simulink model "MS_CDM_substructure"  (R2022b)
settings: Solver=FixedStepAuto  StartTime=0.0  StopTime=55.0  FixedStep=0.001  RelTol=1e-3
values from neighbouring files (symbols this model uses):
  a_ps = K_ps - (2 * M_ps) / (dt)^2    (= -21398788.6)    [Final_10DOFs_RTHS.m]    (also in ThreeDOFs_CDM_substructure.m = -1999400; structure_2DOFs.m = -9.988)
  ACC_el = ACC_el(1:10000,:)    [ThreeDOFs_Dampling.m]    (also in ThreeDOFs_noDampling.m; multiDOFs_CDM_highspeed_Dampling.m = ACC_el(1:2000,:); multiDOFs_auto_for_loop.m = ACC_el(1:1000,:); multiDOFs_highspeed.m = ACC_el(1:1000,:))
  an = Kn - (2 * Mn) / (dt)^2    [Final_10DOFs_RTHS.m]    (also in ThreeDOFs_CDM_Dampling.m; multiDOFs_CDM_highspeed_Dampling.m; test.m)
  b_ps = M_ps / dt^2 - C_ps / (2*dt)    (= 10684932)    [Final_10DOFs_RTHS.m]    (also in ThreeDOFs_CDM_substructure.m = 924875; structure_2DOFs.m = 4)
  bn = Mn / dt^2 - Cn / (2*dt)    [Final_10DOFs_RTHS.m]    (also in ThreeDOFs_CDM_Dampling.m; multiDOFs_CDM_highspeed_Dampling.m; test.m)
  diagM = diag(M)    [CDM_ACC_or_Disp_Input.m]    (also in Final_10DOFs_RTHS.m; ThreeDOFs_CDM_Dampling.m; ThreeDOFs_CDM_substructure.m; ThreeDOFs_Dampling.m)
  dt = 0.001    [CDM_ACC_or_Disp_Input.m]    (also in Final_10DOFs_RTHS.m; ThreeDOFs_CDM_Dampling.m; ThreeDOFs_CDM_substructure.m; ThreeDOFs_Dampling.m)
  Ke_ps_inv = inv(Ke_ps)    [Final_10DOFs_RTHS.m]
  Ken_inv = inv(Ken)    [Final_10DOFs_RTHS.m]
  M_ps = m9 * 1e-5    (= 10.7)    [Final_10DOFs_RTHS.m]    (also in ThreeDOFs_CDM_substructure.m = 1; structure_2DOFs.m = 5e-06)
  ps_weizhi = zeros(length(M_ns),1)    [Final_10DOFs_RTHS.m]
  VV = V(:,1:length(M))    [Final_10DOFs_RTHS.m]    (also in ThreeDOFs_CDM_Dampling.m = V(:,1:3); ThreeDOFs_Dampling.m = V(:,1:3); ThreeDOFs_noDampling.m = V(:,1:3); code.m = V(:,1:3))
libraries: dspsrcs4 x2
settings Model: Creator=dongxh  LastModifiedBy=dongxh

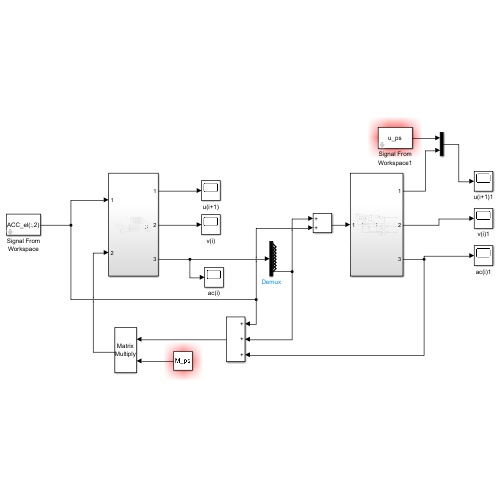
[thumbnail: Simulink's stored preview of the top-level diagram]
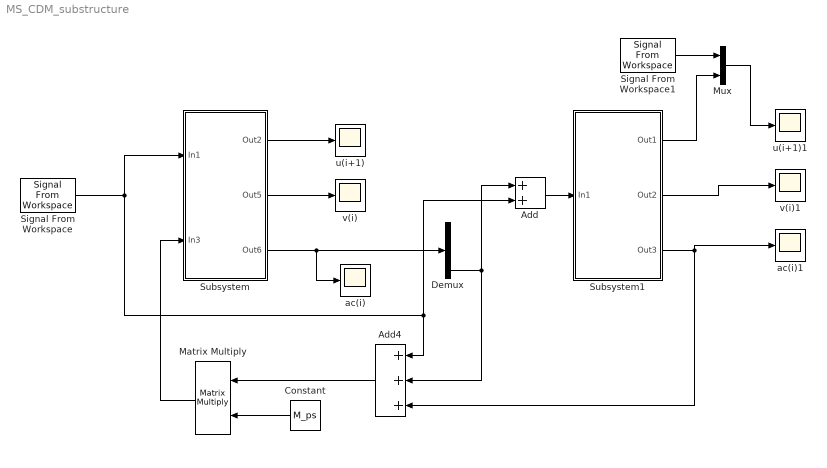
== system MS_CDM_substructure ==
  Add : Sum
  Add4 : Sum  Inputs=+++
  Constant : Constant  Value=M_ps
  Demux : Demux  Outputs=9
  Matrix Multiply : Product  Multiplication=Matrix(*)
  Mux : Mux  Inputs=2
  Signal From Workspace : dspsrcs4/Signal From Workspace  X=ACC_el(:,2)  Ts=0.001  nsamps=1  OutputAfterFinalValue=Setting to zero  ignoreOrWarnInputAndFrameLengths=off  OutputFrames=off
  Signal From Workspace1 : dspsrcs4/Signal From Workspace  X=u_ps  Ts=0.001  nsamps=1  OutputAfterFinalValue=Setting to zero  ignoreOrWarnInputAndFrameLengths=off  OutputFrames=off
  Subsystem : Subsystem
  Subsystem1 : Subsystem
  ac(i) : Scope
  ac(i)1 : Scope
  u(i+1) : Scope
  u(i+1)1 : Scope
  v(i) : Scope
  v(i)1 : Scope
  wires:
  Signal From Workspace/1 -> Add4/1, Add/2, Subsystem/1(In1)
  Subsystem/2(Out5) -> v(i)/1
  Subsystem/3(Out6) -> Demux/1, ac(i)/1
  Subsystem1/3(Out3) -> ac(i)1/1, Add4/3
  Add/1 -> Subsystem1/1(In1)
  Subsystem1/2(Out2) -> v(i)1/1
  Add4/1 -> Matrix Multiply/1
  Constant/1 -> Matrix Multiply/2
  Subsystem1/1(Out1) -> Mux/2
  Mux/1 -> u(i+1)1/1
  Signal From Workspace1/1 -> Mux/1
  Subsystem/1(Out2) -> u(i+1)/1
  Matrix Multiply/1 -> Subsystem/2(In3)
  Demux/9 -> Add4/2, Add/1

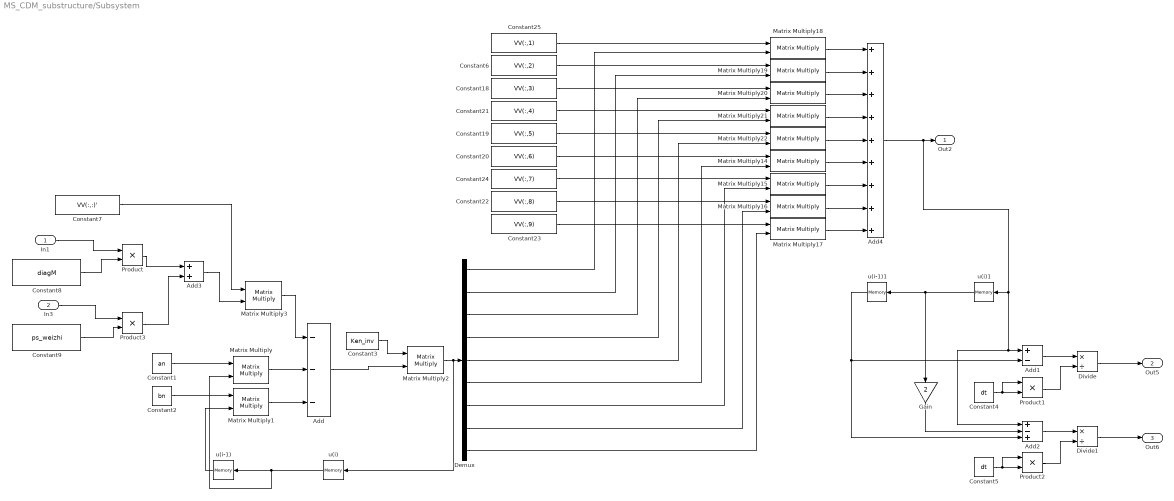
== system MS_CDM_substructure/Subsystem ==
  In1 : Inport
  In3 : Inport  Port=2
  Add : Sum  Inputs=---
  Add1 : Sum  Inputs=+-
  Add2 : Sum  Inputs=+-+
  Add3 : Sum
  Add4 : Sum  Inputs=+++++++++
  Constant1 : Constant  Value=an  VectorParams1D=off
  Constant18 : Constant  Value=VV(:,3)  VectorParams1D=off
  Constant19 : Constant  Value=VV(:,5)  VectorParams1D=off
  Constant2 : Constant  Value=bn  VectorParams1D=off
  Constant20 : Constant  Value=VV(:,6)  VectorParams1D=off
  Constant21 : Constant  Value=VV(:,4)  VectorParams1D=off
  Constant22 : Constant  Value=VV(:,8)  VectorParams1D=off
  Constant23 : Constant  Value=VV(:,9)  VectorParams1D=off
  Constant24 : Constant  Value=VV(:,7)  VectorParams1D=off
  Constant25 : Constant  Value=VV(:,1)  VectorParams1D=off
  Constant3 : Constant  Value=Ken_inv  VectorParams1D=off
  Constant4 : Constant  Value=dt  VectorParams1D=off
  Constant5 : Constant  Value=dt  VectorParams1D=off
  Constant6 : Constant  Value=VV(:,2)  VectorParams1D=off
  Constant7 : Constant  Value=VV(:,:)'  VectorParams1D=off
  Constant8 : Constant  Value=diagM  VectorParams1D=off
  Constant9 : Constant  Value=ps_weizhi  VectorParams1D=off
  Demux : Demux  Outputs=9
  Divide : Product  Inputs=*/
  Divide1 : Product  Inputs=*/
  Gain : Gain  Gain=2
  Matrix Multiply{,1..3,14..22} (13 alike) : Product  Multiplication=Matrix(*)
  Product{,1..3} (4 alike) : Product
  u(i) : Memory
  u(i)1 : Memory
  u(i-1) : Memory
  u(i-1)1 : Memory
  Out2 : Outport
  Out5 : Outport  Port=2
  Out6 : Outport  Port=3
  wires:
  u(i-1)/1 -> Matrix Multiply1/2
  u(i)/1 -> u(i-1)/1, Matrix Multiply/2
  Add/1 -> Matrix Multiply2/2
  Constant1/1 -> Matrix Multiply/1
  Add2/1 -> Divide1/1
  Constant5/1 -> Product2/2, Product2/1
  Matrix Multiply2/1 -> Demux/1, u(i)/1
  Constant4/1 -> Product1/1, Product1/2
  Gain/1 -> Add2/2
  Product1/1 -> Divide/2
  Constant2/1 -> Matrix Multiply1/1
  Constant3/1 -> Matrix Multiply2/1
  Add1/1 -> Divide/1
  Divide1/1 -> Out6/1
  Product2/1 -> Divide1/2
  Divide/1 -> Out5/1
  In1/1 -> Product/1
  Constant8/1 -> Product/2
  Product/1 -> Add3/1
  Product3/1 -> Add3/2
  In3/1 -> Product3/1
  Constant9/1 -> Product3/2
  Matrix Multiply1/1 -> Add/3
  Matrix Multiply/1 -> Add/2
  Matrix Multiply3/1 -> Add/1
  Demux/1 -> Matrix Multiply18/2
  Demux/2 -> Matrix Multiply19/2
  Demux/3 -> Matrix Multiply20/2
  Demux/4 -> Matrix Multiply21/2
  Demux/5 -> Matrix Multiply22/2
  Demux/6 -> Matrix Multiply14/2
  Demux/7 -> Matrix Multiply15/2
  Demux/8 -> Matrix Multiply16/2
  Demux/9 -> Matrix Multiply17/2
  Matrix Multiply18/1 -> Add4/1
  Matrix Multiply19/1 -> Add4/2
  Matrix Multiply20/1 -> Add4/3
  Matrix Multiply21/1 -> Add4/4
  Matrix Multiply22/1 -> Add4/5
  Matrix Multiply14/1 -> Add4/6
  Matrix Multiply15/1 -> Add4/7
  Matrix Multiply16/1 -> Add4/8
  Matrix Multiply17/1 -> Add4/9
  Add4/1 -> Add2/1, Add1/1, u(i)1/1, Out2/1
  Constant7/1 -> Matrix Multiply3/1
  Add3/1 -> Matrix Multiply3/2
  Constant25/1 -> Matrix Multiply18/1
  Constant6/1 -> Matrix Multiply19/1
  Constant18/1 -> Matrix Multiply20/1
  Constant21/1 -> Matrix Multiply21/1
  Constant19/1 -> Matrix Multiply22/1
  Constant20/1 -> Matrix Multiply14/1
  Constant24/1 -> Matrix Multiply15/1
  Constant22/1 -> Matrix Multiply16/1
  Constant23/1 -> Matrix Multiply17/1
  u(i)1/1 -> Gain/1, u(i-1)1/1
  u(i-1)1/1 -> Add2/3, Add1/2

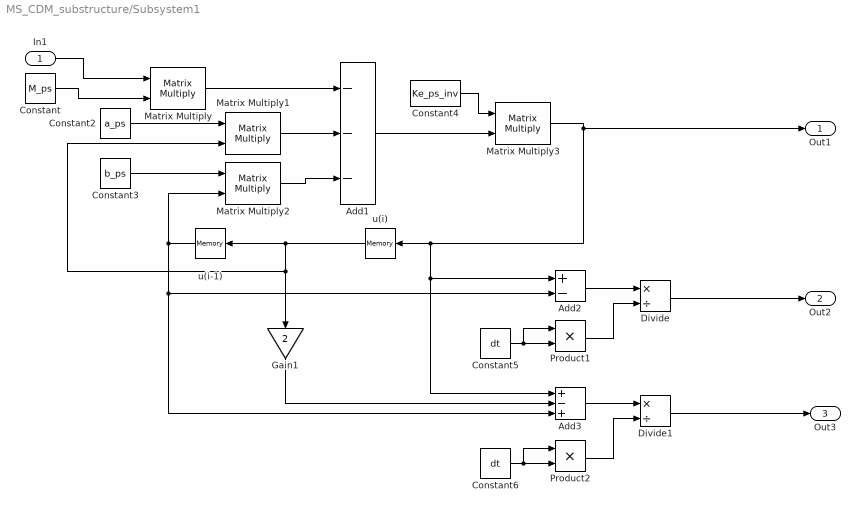
== system MS_CDM_substructure/Subsystem1 ==
  In1 : Inport
  Add1 : Sum  Inputs=---
  Add2 : Sum  Inputs=+-
  Add3 : Sum  Inputs=+-+
  Constant : Constant  Value=M_ps
  Constant2 : Constant  Value=a_ps  VectorParams1D=off
  Constant3 : Constant  Value=b_ps  VectorParams1D=off
  Constant4 : Constant  Value=Ke_ps_inv  VectorParams1D=off
  Constant5 : Constant  Value=dt  VectorParams1D=off
  Constant6 : Constant  Value=dt  VectorParams1D=off
  Divide : Product  Inputs=*/
  Divide1 : Product  Inputs=*/
  Gain1 : Gain  Gain=2
  Matrix Multiply{,1..3} (4 alike) : Product  Multiplication=Matrix(*)
  Product1 : Product
  Product2 : Product
  u(i) : Memory
  u(i-1) : Memory
  Out1 : Outport
  Out2 : Outport  Port=2
  Out3 : Outport  Port=3
  wires:
  Matrix Multiply1/1 -> Add1/2
  Matrix Multiply/1 -> Add1/1
  Matrix Multiply3/1 -> Out1/1, Add3/1, Add2/1, u(i)/1
  Product2/1 -> Divide1/2
  Constant/1 -> Matrix Multiply/2
  u(i-1)/1 -> Matrix Multiply2/2, Add3/3, Add2/2
  Product1/1 -> Divide/2
  Constant3/1 -> Matrix Multiply2/1
  In1/1 -> Matrix Multiply/1
  u(i)/1 -> u(i-1)/1, Matrix Multiply1/2, Gain1/1
  Constant5/1 -> Product1/1, Product1/2
  Add2/1 -> Divide/1
  Constant4/1 -> Matrix Multiply3/1
  Constant6/1 -> Product2/2, Product2/1
  Constant2/1 -> Matrix Multiply1/1
  Gain1/1 -> Add3/2
  Add1/1 -> Matrix Multiply3/2
  Add3/1 -> Divide1/1
  Matrix Multiply2/1 -> Add1/3
  Divide1/1 -> Out3/1
  Divide/1 -> Out2/1
